simulink model "lqr_nonlinear"  (R2022a)
settings: Solver=VariableStepAuto  StartTime=0.0  StopTime=20  RelTol=1e-3
undefined symbols (not defined in the file or in its folder): g, K_d, l, m, M, Ts
settings Model: Creator=uzivatel  LastModifiedBy=uzivatel

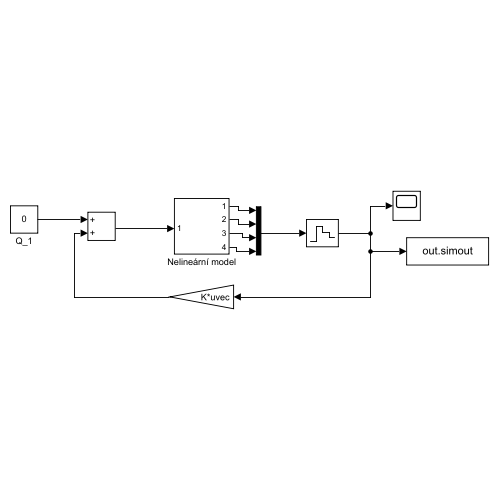
[thumbnail: Simulink's stored preview of the top-level diagram]
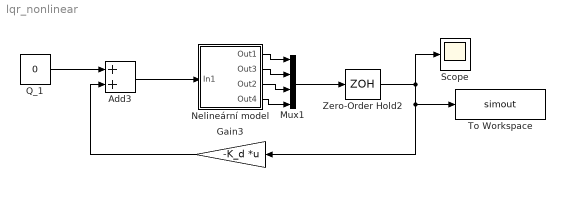
== system lqr_nonlinear ==
  Add3 : Sum
  Gain3 : Gain  Gain=-K_d  Multiplication=Matrix(K*u) (u vector)
  Mux1 : Mux
  Nelineární model : Subsystem
  Q_1 : Constant  Value=0
  Scope : Scope
  To Workspace : ToWorkspace  VariableName=simout  SaveFormat=Timeseries  SampleTime=-1
  Zero-Order Hold2 : ZeroOrderHold  SampleTime=Ts
  wires:
  Nelineární model/4(Out4) -> Mux1/4
  Mux1/1 -> Zero-Order Hold2/1
  Q_1/1 -> Add3/1
  Nelineární model/2(Out3) -> Mux1/2
  Gain3/1 -> Add3/2
  Nelineární model/1(Out1) -> Mux1/1
  Nelineární model/3(Out2) -> Mux1/3
  Zero-Order Hold2/1 -> To Workspace/1, Gain3/1, Scope/1
  Add3/1 -> Nelineární model/1(In1)

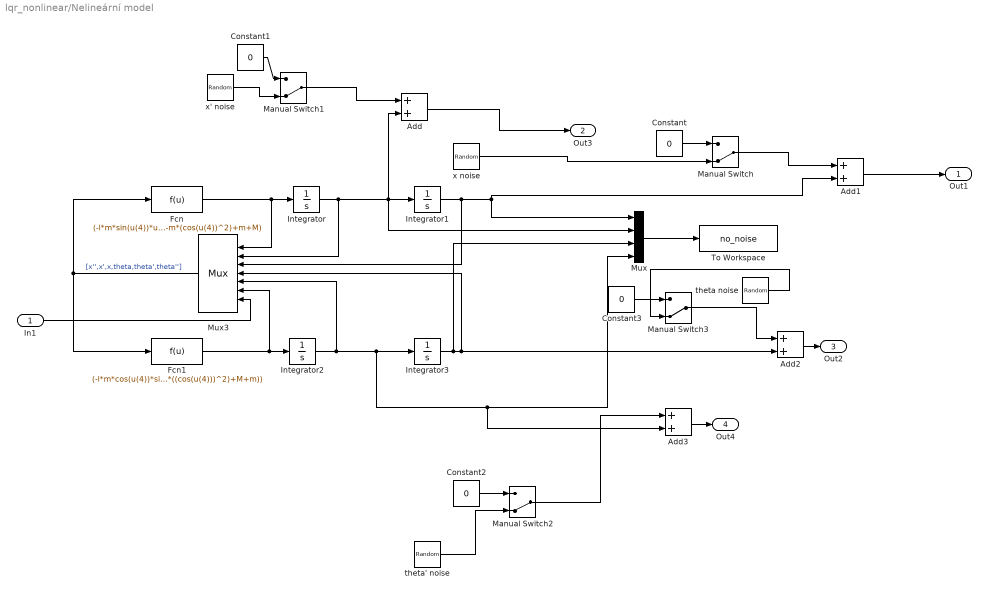
== system lqr_nonlinear/Nelineární model ==
  In1 : Inport
  Add{,1..3} (4 alike) : Sum
  Constant{,1..3} (4 alike) : Constant  Value=0
  Fcn : Fcn  Expr=(-l*m*sin(u(4))*u(5)^2+u(7)-m*g*cos(u(4))*sin(u(4)))/(-m*(cos(u(4))^2)+m+M)
  Fcn1 : Fcn  Expr=(-l*m*cos(u(4))*sin(u(4))*u(5)^2+u(7)*cos(u(4))-g*m*sin(u(4))-M*g*sin(u(4)))/(l*(-m*((cos(u(4)))^2)+M+m))
  Integrator : Integrator
  Integrator1 : Integrator
  Integrator2 : Integrator
  Integrator3 : Integrator  InitialCondition=pi/6
  Manual Switch{,1..3} (4 alike) : ManualSwitch  CurrentSetting=0
  Mux : Mux
  Mux3 : Mux  Inputs=7
      settings: DisplayOption=signals
  To Workspace : ToWorkspace  VariableName=no_noise  SaveFormat=Timeseries  SampleTime=-1
  theta noise : RandomNumber  Variance=0.05^2  SampleTime=0.033
  theta' noise : RandomNumber  Variance=0.02^2  SampleTime=0.033
  x noise : RandomNumber  Variance=0.1^2  SampleTime=0.033
  x' noise : RandomNumber  Variance=0.02^2  SampleTime=0.033
  Out1 : Outport
  Out3 : Outport  Port=2
  Out2 : Outport  Port=3
  Out4 : Outport  Port=4
  wires:
  Integrator/1 -> Mux/2, Add/2, Integrator1/1, Mux3/2
  Fcn1/1 -> Mux3/6, Integrator2/1
  Mux3/1 -> Fcn/1, Fcn1/1  "[x'',x',x,theta,theta',theta'']"
  Integrator1/1 -> Mux/1, Add1/2, Mux3/3
  Integrator3/1 -> Mux/3, Add2/2, Mux3/4
  Integrator2/1 -> Mux3/5, Mux/4, Add3/2, Integrator3/1
  Fcn/1 -> Mux3/1, Integrator/1
  In1/1 -> Mux3/7
  Add/1 -> Out3/1
  x noise/1 -> Manual Switch/2
  Add1/1 -> Out1/1
  Add2/1 -> Out2/1
  Add3/1 -> Out4/1
  Mux/1 -> To Workspace/1
  Constant/1 -> Manual Switch/1
  Manual Switch/1 -> Add1/1
  Constant1/1 -> Manual Switch1/1
  Manual Switch1/1 -> Add/1
  x' noise/1 -> Manual Switch1/2
  Constant2/1 -> Manual Switch2/1
  Manual Switch2/1 -> Add3/1
  theta' noise/1 -> Manual Switch2/2
  Constant3/1 -> Manual Switch3/1
  Manual Switch3/1 -> Add2/1
  theta noise/1 -> Manual Switch3/2
